simulink model "MicrowaveV2_2015a"  (Simulink 8.5)
settings: Solver=FixedStepDiscrete  StartTime=0.0  StopTime=20  RelTol=1e-3
libraries: simulink x1
settings Model: Creator=bourbouh  LastModifiedBy=hamza
settings DataIOCC: SaveFormat=Dataset  SignalLoggingSaveFormat=Dataset  SaveOutput=off  SignalLogging=off  DSMLogging=off  SaveTime=off
settings OptimizationCC: ExpressionDepthLimit=128
settings DebuggingCC: UnderspecifiedInitializationDetection=Simplified  MergeDetectMultiDrivingBlocksExec=error  FcnCallInpInsideContextMsg=EnableAllAsError  StateNameClashWarn=none
settings GRTTargetCC: CombineOutputUpdateFcns=on  GRTInterface=off

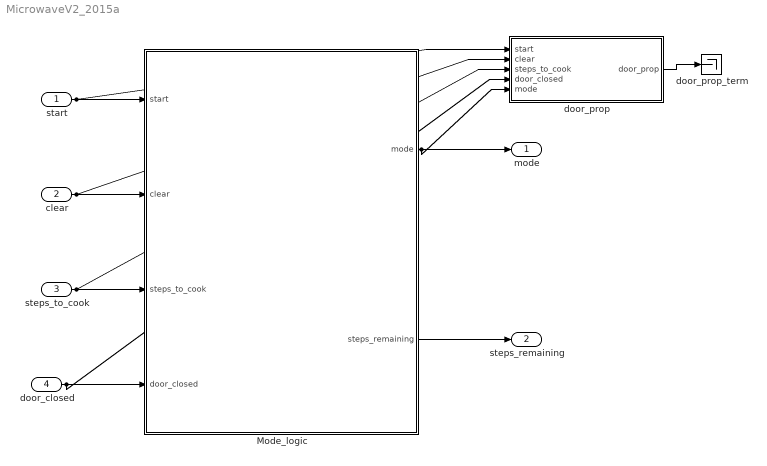
== system MicrowaveV2_2015a ==
  start : Inport
  clear : Inport  Port=2
  steps_to_cook : Inport  Port=3
  door_closed : Inport  Port=4
  Mode_logic : Stateflow chart  TreatAsAtomicUnit=on
      settings: PermitHierarchicalResolution=ParametersOnly
  door_prop : Subsystem  TreatAsAtomicUnit=on  mask(Observer){AnnotationType=ensures, ObserverType=[]}
      mask prompts: AnnotationType "Type of annotation (pre/post...)"; ObserverType "Observer type"
      mask help:
      | Set an observer for the system.
      | The annotation type parameter sets the type of observer:
      | - requires : pre-condition
      | - ensures : post-condition
      | - assert : an assertion
      | - observer : the observer computes a special type of properties
      mask TypeOptions AnnotationType: ensures | requires | assert | observer
      mask Callback AnnotationType:
      | paramStr = get_param(gcb, 'MaskValues');
      | if strcmp(paramStr{1}(1),'o')
      | set_param(gcb,'MaskVisibilities',{'on';'on'});
      | paramStr{2} = 'ellipsoid';
      | set_param(gcb,'MaskValues',paramStr);
      | else
      | set_param(gcb,'MaskVisibilities',{'on';'off'});
      | end
      | clear paramStr;
      mask Callback ObserverType:
      | paramStr = get_param(gcb, 'MaskValues');
      | if strcmp(paramStr{1}(1),'o')
      | set_param(gcb,'MaskVisibilities',{'on';'on'});
      | paramStr{2} = 'ellipsoid';
      | set_param(gcb,'MaskValues',paramStr);
      | else
      | set_param(gcb,'MaskVisibilities',{'on';'off'});
      | end
      | clear paramStr;
      mask Display:
      | color('black')
      | text(0.5, 0.5, ['Property: ''' get_param(gcb,'name') ''''], 'horizontalAlignment', 'center');
      | text(0.99, 0.03, '{\bf\fontsize{12}SAFE}', 'hor', 'right', 'ver', 'bottom', 'texmode', 'on');
  door_prop_term : Terminator
  mode : Outport
  steps_remaining : Outport  Port=2
  wires:
  start/1 -> Mode_logic/1(start), door_prop/1(start)
  door_closed/1 -> door_prop/4(door_closed), Mode_logic/4(door_closed)
  steps_to_cook/1 -> Mode_logic/3(steps_to_cook), door_prop/3(steps_to_cook)
  clear/1 -> Mode_logic/2(clear), door_prop/2(clear)
  Mode_logic/1(mode) -> door_prop/5(mode), mode/1
  Mode_logic/2(steps_remaining) -> steps_remaining/1
  door_prop/1(door_prop) -> door_prop_term/1

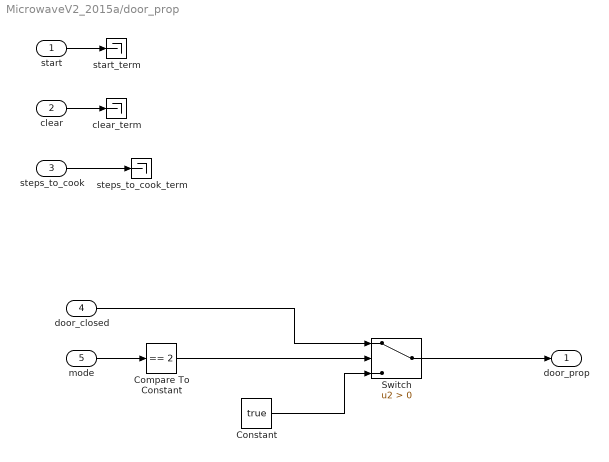
== system MicrowaveV2_2015a/door_prop ==
  start : Inport
  clear : Inport  Port=2
  steps_to_cook : Inport  Port=3
  door_closed : Inport  Port=4
  mode : Inport  Port=5
  Compare To Constant : simulink/Logic and Bit Operations/Compare To Constant  relop===  const=2  OutDataTypeStr=boolean
  Constant : Constant  Value=true
  Switch : Switch  Criteria=u2 > Threshold
  clear_term : Terminator
  start_term : Terminator
  steps_to_cook_term : Terminator
  door_prop : Outport
  wires:
  start/1 -> start_term/1
  clear/1 -> clear_term/1
  steps_to_cook/1 -> steps_to_cook_term/1
  door_closed/1 -> Switch/1
  Switch/1 -> door_prop/1
  Constant/1 -> Switch/3
  mode/1 -> Compare To Constant/1
  Compare To Constant/1 -> Switch/2

== stateflow chart Mode_logic ==
  settings: updateMethod=DISCRETE  sampleTime=1
  state SETUP
    entry:
    mode=1;
    steps_remaining = steps_to_cook;
  state RUNNING
    state COOKING
      entry: mode=2;
    state SUSPENDED
      entry: mode=3;
    COOKING -> COOKING [order 2] : [steps_remaining > 0]
        | /steps_remaining--;
    (default) -> (junction 7)
    (junction 7) -> COOKING [order 1] : [door_closed]
    (junction 7) -> SUSPENDED [order 2]
    SUSPENDED -> COOKING [order 2] : [start && ...
        | door_closed]
    COOKING -> SUSPENDED [order 1] : [clear || ...
        | !door_closed]
  (default) -> SETUP
  SETUP -> RUNNING : [start && steps_to_cook > 0]{steps_remaining = steps_to_cook;}
  (junction 20) -> SETUP
  RUNNING -> (junction 20) : [steps_remaining <= 0]
  SUSPENDED -> (junction 20) [order 1] : [clear]
  data: start input boolean; clear input boolean; steps_to_cook input uint16; door_closed input boolean; mode output uint8; steps_remaining output uint16 [0..600]
